simulink model "CRC_example"  (R2022a)
settings: Solver=VariableStepAuto  StartTime=0.0  StopTime=60  RelTol=1e-3
libraries: dspsrcs4 x4, whdledac x1, whdlutilities x1, xilinxrfsoclib x1
settings Model: Creator=Zeyan Wu  LastModifiedBy=Zeyan Wu

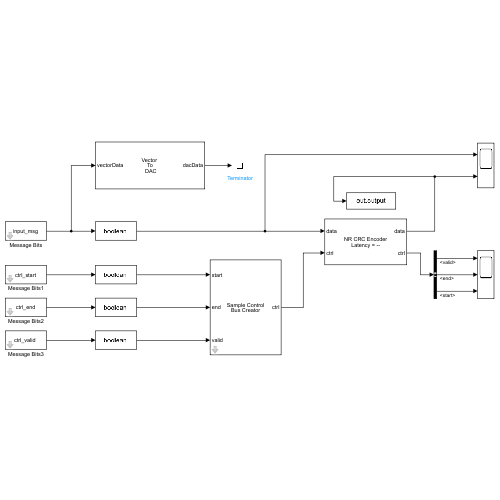
[thumbnail: Simulink's stored preview of the top-level diagram]
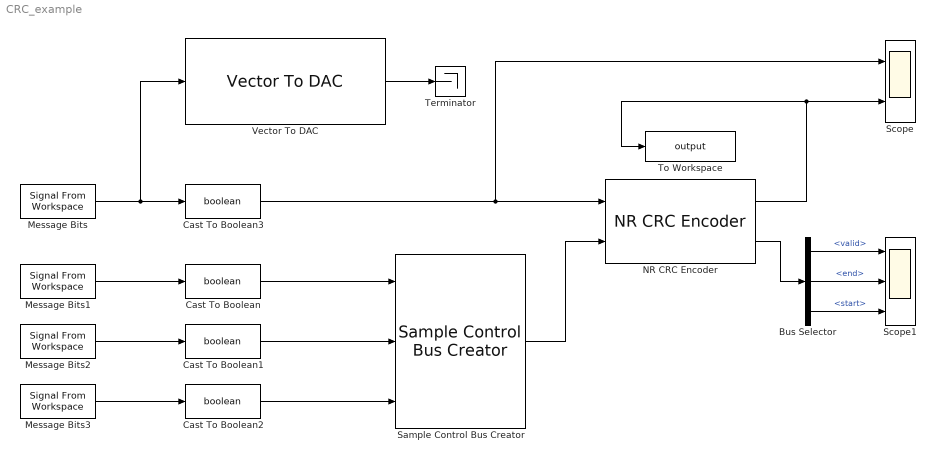
== system CRC_example ==
  Bus Selector : BusSelector  OutputSignals=valid,end,start
  Cast To Boolean{,1..3} (4 alike) : DataTypeConversion  OutDataTypeStr=boolean  SaturateOnIntegerOverflow=off  RndMeth=Floor
  Message Bits : dspsrcs4/Signal From Workspace  X=input_msg  Ts=1  nsamps=1  OutputAfterFinalValue=Setting to zero  ignoreOrWarnInputAndFrameLengths=off  OutputFrames=on
  Message Bits1 : dspsrcs4/Signal From Workspace  X=ctrl_start  Ts=1  nsamps=1  OutputAfterFinalValue=Setting to zero  ignoreOrWarnInputAndFrameLengths=off  OutputFrames=on
  Message Bits2 : dspsrcs4/Signal From Workspace  X=ctrl_end  Ts=1  nsamps=1  OutputAfterFinalValue=Setting to zero  ignoreOrWarnInputAndFrameLengths=off  OutputFrames=on
  Message Bits3 : dspsrcs4/Signal From Workspace  X=ctrl_valid  Ts=1  nsamps=1  OutputAfterFinalValue=Setting to zero  ignoreOrWarnInputAndFrameLengths=off  OutputFrames=on
  NR CRC Encoder : whdledac/NR CRC Encoder  CRCType=CRC16  EnableCRCMaskPort=off  SimulateUsing=Code generation
      settings: SourceProductBaseCode=LH
  Sample Control Bus Creator : whdlutilities/Sample Control Bus Creator
      settings: SourceProductBaseCode=LH
  Scope : Scope  NumInputPorts=2
  Scope1 : Scope  NumInputPorts=3
  Terminator : Terminator
  To Workspace : ToWorkspace  VariableName=output  SampleTime=1
      settings: Save2DSignal=2-D array (concatenate along first dimension)
  Vector To DAC : xilinxrfsoclib/Vector To DAC  INPUT_WL=16  DT_INPUT=0
      settings: SourceProductBaseCode=XILINX_BLOCKSET
  wires:
  Message Bits2/1 -> Cast To Boolean1/1
  Message Bits1/1 -> Cast To Boolean/1
  Message Bits3/1 -> Cast To Boolean2/1
  Sample Control Bus Creator/1 -> NR CRC Encoder/2
  Cast To Boolean/1 -> Sample Control Bus Creator/1
  Cast To Boolean1/1 -> Sample Control Bus Creator/2
  Cast To Boolean2/1 -> Sample Control Bus Creator/3
  NR CRC Encoder/2 -> Bus Selector/1
  Bus Selector/1 -> Scope1/1  "<valid>"
  Bus Selector/3 -> Scope1/3  "<start>"
  NR CRC Encoder/1 -> Scope/2, To Workspace/1
  Bus Selector/2 -> Scope1/2  "<end>"
  Message Bits/1 -> Cast To Boolean3/1, Vector To DAC/1
  Cast To Boolean3/1 -> Scope/1, NR CRC Encoder/1
  Vector To DAC/1 -> Terminator/1
